simulink model "chi_reference"  (R2016a)
settings: Solver=VariableStepAuto  StartTime=0.0  StopTime=total_time  RelTol=1e-3
values from neighbouring files (symbols this model uses):
  angle1 = deg2rad(5)    [Copy_of_modelParms.m]    (also in modelParms.m)
  angle2 = deg2rad(-5)    [Copy_of_modelParms.m]    (also in modelParms.m)
  angle3 = deg2rad(15)    [Copy_of_modelParms.m]    (also in modelParms.m)
  angle4 = deg2rad(-20)    [Copy_of_modelParms.m]    (also in modelParms.m)
  t1 = 100    [Copy_of_modelParms.m]    (also in modelParms.m)
  t2 = t1+100    (= 200)    [Copy_of_modelParms.m]    (also in modelParms.m)
  t3 = t2+100    (= 300)    [Copy_of_modelParms.m]    (also in modelParms.m)
settings Model: Creator=Alex  LastModifiedBy=Alex

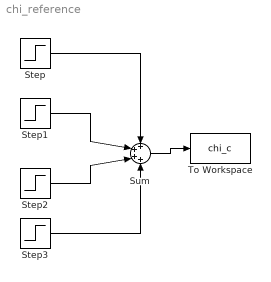
== system chi_reference ==
  Step : Step  Time=0  After=angle1  SampleTime=0
  Step1 : Step  Time=t1  After=angle2  SampleTime=0
  Step2 : Step  Time=t2  After=angle3  SampleTime=0
  Step3 : Step  Time=t3  After=angle4  SampleTime=0
  Sum : Sum  Inputs=++++
  To Workspace : ToWorkspace  VariableName=chi_c  SaveFormat=Timeseries  SampleTime=-1
  wires:
  Step/1 -> Sum/1
  Sum/1 -> To Workspace/1
  Step1/1 -> Sum/2
  Step2/1 -> Sum/3
  Step3/1 -> Sum/4
